simulink model "TD1"  (R2024b)
settings: Solver=VariableStepAuto  StartTime=0.0  StopTime=200  RelTol=1e-3
libraries: slpidlib x1
settings Model: Creator=simon  LastModifiedBy=simon

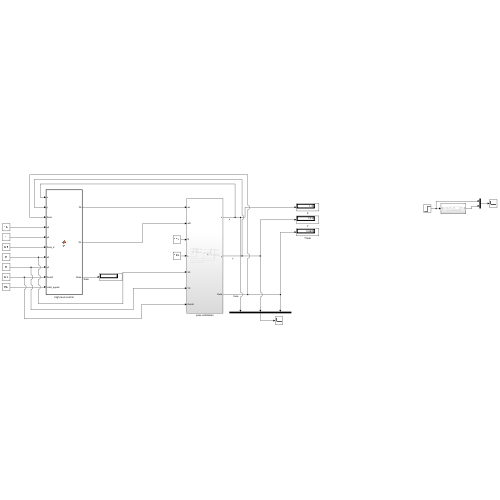
[thumbnail: Simulink's stored preview of the top-level diagram]
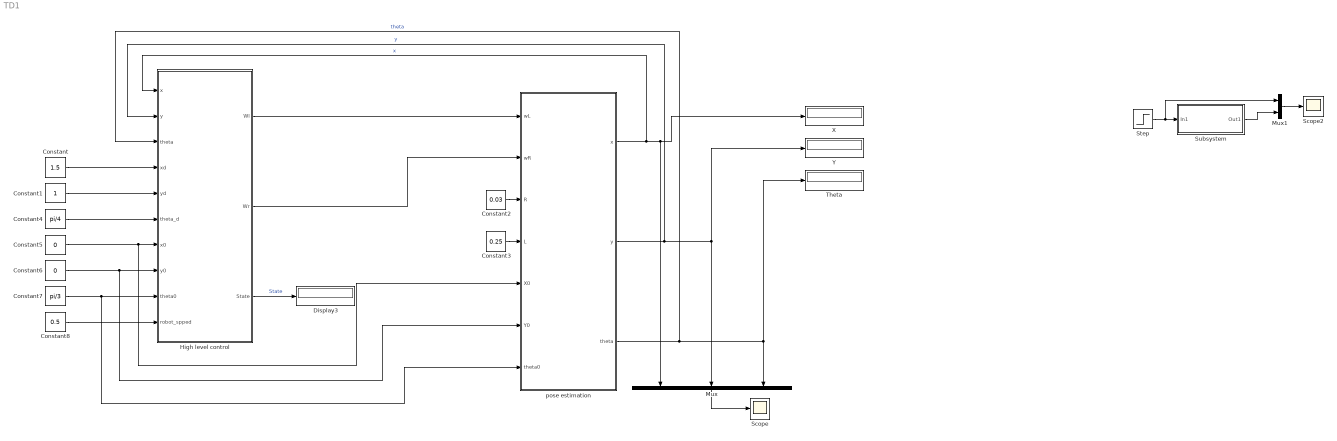
== system TD1 ==
  Constant : Constant  Value=1.5
  Constant1 : Constant
  Constant2 : Constant  Value=0.03
  Constant3 : Constant  Value=0.25
  Constant4 : Constant  Value=pi/4
  Constant5 : Constant  Value=0
  Constant6 : Constant  Value=0
  Constant7 : Constant  Value=pi/3
  Constant8 : Constant  Value=0.5
  Display3 : Display
  High level control : MATLAB Function  TreatAsAtomicUnit=on
  Mux : Mux  Inputs=3
  Mux1 : Mux  Inputs=2
  Scope : Scope
  Scope2 : Scope
  Step : Step  SampleTime=1
  Subsystem : Subsystem
  Theta : Display
  X : Display
  Y : Display
  pose estimation : Subsystem
  wires:
  pose estimation/1(x) -> X/1, Mux/1, High level control/1(x)  "x"
  pose estimation/2(y) -> High level control/2(y), Y/1, Mux/2  "y"
  pose estimation/3(theta) -> Theta/1, Mux/3, High level control/3(theta)  "theta"
  Mux/1 -> Scope/1
  Constant2/1 -> pose estimation/3(R)
  Constant3/1 -> pose estimation/4(L)
  Constant/1 -> High level control/4(xd)
  Constant1/1 -> High level control/5(yd)
  Constant4/1 -> High level control/6(theta_d)
  Constant5/1 -> pose estimation/5(X0), High level control/7(x0)
  Constant6/1 -> High level control/8(y0), pose estimation/6(Y0)
  Constant7/1 -> pose estimation/7(theta0), High level control/9(theta0)
  Constant8/1 -> High level control/10(robot_spped)
  High level control/2(Wr) -> pose estimation/2(wR)
  High level control/1(Wl) -> pose estimation/1(wL)
  High level control/3(State) -> Display3/1  "State"
  Subsystem/1(Out1) -> Mux1/2
  Step/1 -> Subsystem/1(In1), Mux1/1
  Mux1/1 -> Scope2/1

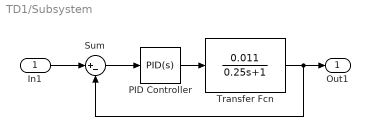
== system TD1/Subsystem ==
  In1 : Inport
  PID Controller : slpidlib/PID Controller  Controller=PID  Form=Parallel  TimeDomain=Continuous-time  UseExternalTs=off  SampleTime=-1  IntegratorMethod=Forward Euler  FilterMethod=Forward Euler  ControllerParametersSource=internal  P=80  I=400  UseKiTs=off  D=0  UseExternalDerivativeSource=off  N=100  UseFilter=on  TunerSelectOption=Transfer Function Based (PID Tuner App)  InitialConditionSource=internal  InitialConditionForIntegrator=0  InitialConditionForFilter=0  DifferentiatorICPrevScaledInput=0  ExternalReset=none  TrackingMode=off  Kt=1  LimitOutput=off  SatLimitsSource=internal  UpperSaturationLimit=inf  LowerSaturationLimit=-inf  LinearizeAsGain=on  AntiWindupMode=none  Kb=1  LimitIntegrator=off  UpperIntegratorSaturationLimit=inf  LowerIntegratorSaturationLimit=-inf  POutMin=[]  POutMax=[]  IOutMin=[]  IOutMax=[]  DOutMin=[]  DOutMax=[]  NOutMin=[]  NOutMax=[]  SumOutMin=[]  SumOutMax=[]  SaturationOutMin=[]  SaturationOutMax=[]  PParamMin=[]  PParamMax=[]  IParamMin=[]  IParamMax=[]  DParamMin=[]  DParamMax=[]  NParamMin=[]  NParamMax=[]  KbParamMin=[]  KbParamMax=[]  KtParamMin=[]  KtParamMax=[]  KbOutMin=[]  KbOutMax=[]  KtOutMin=[]  KtOutMax=[]  IntegratorOutMin=[]  IntegratorOutMax=[]  FilterOutMin=[]  FilterOutMax=[]  SumI1OutMin=[]  SumI1OutMax=[]  SumI2OutMin=[]  SumI2OutMax=[]  SumI3OutMin=[]  SumI3OutMax=[]  SumI4OutMin=[]  SumI4OutMax=[]  SumDOutMin=[]  SumDOutMax=[]  DifferentiatorOutMin=[]  DifferentiatorOutMax=[]  FilterDiffOutCoefMin=[]  FilterDiffOutCoefMax=[]  ReciprocalOutMin=[]  ReciprocalOutMax=[]  SumDenOutMin=[]  SumDenOutMax=[]  SumNumOutMin=[]  SumNumOutMax=[]  DivideOutMin=[]  DivideOutMax=[]  UdiffTsProdOutMin=[]  UdiffTsProdOutMax=[]  NTsProdOutMin=[]  NTsProdOutMax=[]  UintegralTsProdOutMin=[]  UintegralTsProdOutMax=[]  UngainTsProdOutMin=[]  UngainTsProdOutMax=[]  ClampingZeroOutDataTypeStr=Inherit: Inherit via back propagation  ClampingZeroOutMin=[]  ClampingZeroOutMax=[]  FilterDenConstantOutDataTypeStr=Inherit: Inherit via back propagation  FilterDenConstantOutMin=[]  FilterDenConstantOutMax=[]  PCopyOutDataTypeStr=Inherit: Inherit via back propagation  PCopyOutMin=[]  PCopyOutMax=[]  NCopyOutDataTypeStr=Inherit: Inherit via back propagation  NCopyOutMin=[]  NCopyOutMax=[]  IntegratorContinuousStateAttributes=''  IntegratorStateMustResolveToSignalObject=off  IntegratorRTWStateStorageClass=Auto  FilterContinuousStateAttributes=''  FilterStateMustResolveToSignalObject=off  FilterRTWStateStorageClass=Auto  ParallelPVariant=InternalParameters  IdealPVariant=Disabled  IVariant=InternalParameters  DVariant=InternalParameters  IntegratorVariant=Continuous  SatVariant=Disabled  AWVariant=Passthrough  PCopyVariant=Disabled  TRVariant=Disabled  FdbkBlocksVariant=Forward  IdealPFdbkVariant=Disabled  SatFdbkVariant=Disabled  DerivativeFilterVariant=ContFilter  NVariant=InternalParameters  NCopyVariant=Disabled  FilterICVariant=InternalICsFilter  IntegratorICVariant=InternalICs  ExternalResetVariant=Disabled  TRSumVariant=Passthrough  SumFdbkVariant=Disabled  SumVariant=Sum_PID  TsampFilterVariant=InternalTs  TsampNgainVariant=Passthrough  TsampIntegralVariant=Disabled_SignalSpec  ExternalSaturationOutDataTypeStr=Inherit: Same as second input  DerivativeSourceVariant=ErrorSignal  PreIntVariant=InternalPreInt
  Sum : Sum  Inputs=|+-
  Transfer Fcn : TransferFcn  Numerator=0.011  Denominator=[0.25 1]
  Out1 : Outport
  wires:
  In1/1 -> Sum/1
  Sum/1 -> PID Controller/1
  Transfer Fcn/1 -> Sum/2, Out1/1
  PID Controller/1 -> Transfer Fcn/1

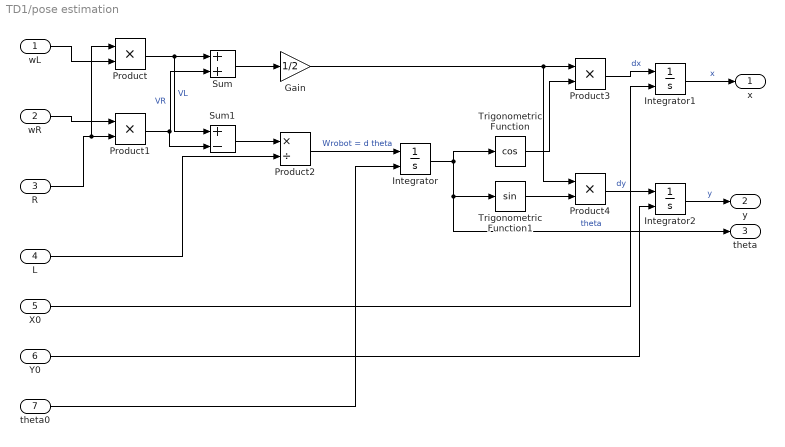
== system TD1/pose estimation ==
  wL : Inport
  wR : Inport  Port=2
  R : Inport  Port=3
  L : Inport  Port=4
  X0 : Inport  Port=5
  Y0 : Inport  Port=6
  theta0 : Inport  Port=7
  Gain : Gain  Gain=1/2
  Integrator : Integrator  InitialConditionSource=external
  Integrator1 : Integrator  InitialConditionSource=external
  Integrator2 : Integrator  InitialConditionSource=external
  Product{,1,3..4} (4 alike) : Product
  Product2 : Product  Inputs=*/
  Sum : Sum
  Sum1 : Sum  Inputs=+-
  Trigonometric Function : Trigonometry  Operator=cos
  Trigonometric Function1 : Trigonometry
  x : Outport
  y : Outport  Port=2
  theta : Outport  Port=3
  wires:
  L/1 -> Product2/2
  Integrator2/1 -> y/1  "y"
  Trigonometric Function/1 -> Product3/2
  Trigonometric Function1/1 -> Product4/2
  Gain/1 -> Product4/1, Product3/1
  Product3/1 -> Integrator1/1  "dx"
  R/1 -> Product/1, Product1/2
  Sum1/1 -> Product2/1
  Product2/1 -> Integrator/1  "Wrobot = d theta"
  Sum/1 -> Gain/1
  Product4/1 -> Integrator2/1  "dy"
  Integrator1/1 -> x/1  "x"
  Integrator/1 -> Trigonometric Function/1, Trigonometric Function1/1, theta/1  "theta"
  Product/1 -> Sum1/1, Sum/1  "VL"
  Product1/1 -> Sum1/2, Sum/2  "VR"
  wL/1 -> Product/2
  wR/1 -> Product1/1
  X0/1 -> Integrator1/2
  Y0/1 -> Integrator2/2
  theta0/1 -> Integrator/2

== matlab function TD1/High level control ==
  data: x input; Wl output; y input; theta input; xd input; yd input; theta_d input; x0 input; y0 input; theta0 input; robot_spped input; Wr output; State output
function [Wl, Wr, State] = fcn(x, y, theta, xd, yd, theta_d, x0, y0, theta0, robot_spped)
% State 0 : Initial condition

% State 4 : Stop the robot
Wl = 0;
Wr = 0;
State = 0;

TD = sqrt((xd-x0).^2+ (yd-y0).^2);
Ta = sqrt((x-x0).^2 + (y-y0).^2); % distance parcourue

theta1 = sign(yd - y0).*acos((xd-x0)/TD)-theta;
theta2 = theta_d - theta;

C1 = theta1 > 0.01 || theta1 < -0.01;
C2 = Ta <= TD;
C3 = theta2 > 0.1 || theta2 < -0.1;


% Calculation of appropriate state
if (C1 && C2) % pour ne pas re-rentrer dans le C1 lors du state 3
    State = 1; % State 1: Rotation of θ1
elseif (C2)
    State = 2; % State 2: Straight line of TD
elseif(C3)
    State = 3; % State 3: Rotation of θ2
else
    State = 4;
end

% Control the robot according to the state
switch State
    case 1
        if (theta1 > 0)
            Wl = robot_spped;
            Wr = -robot_spped;
        else 
            Wl = -robot_spped;
            Wr = robot_spped;
        end

    case 2
        Wl = robot_spped;
        Wr = robot_spped;
    case 3
        if (theta2 > 0)
            Wl = robot_spped;
            Wr = -robot_spped;
        else
            Wl = -robot_spped;
            Wr = robot_spped;
        end

    otherwise
        Wl = 0;
        Wr = 0;
end
